simulink model "fan_Ex5"  (R2023b)
settings: Solver=FixedStepAuto  StartTime=0.0  StopTime=10.0  RelTol=1e-3
settings Model: Creator=Fartash  LastModifiedBy=Fartash
settings OptimizationCC: DefaultParameterBehavior=Inlined  EnhancedBackFolding=on  PassReuseOutputArgsAs=Individual arguments  InitFltsAndDblsToZero=on  OptimizeBlockOrder=speed  DifferentSizesBufferReuse=on  OptimizationCustomize=off  EfficientTunableParamExpr=on
settings DebuggingCC: ParameterTunabilityLossMsg=error
settings HardwareCC: ProdLongLongMode=on  TargetLongLongMode=on
settings SFSimCC: MATLABDynamicMemAlloc=off  SimTargetLang=C++
settings RTWCC: Description=Embedded Coder  SystemTargetFile=ert.tlc  GenCodeOnly=on  TemplateMakefile=ert_default_tmf  Toolchain=MinGW64 | CMake/Ninja (64-bit Windows)  BuildConfiguration=Release  TargetLang=C++  GenerateGPUCode=CUDA
settings CodeAppCC: ForceParamTrailComments=on  IgnoreCustomStorageClasses=off  OperatorAnnotations=on  SimulinkDataObjDesc=on  SFDataObjDesc=on  InsertBlockDesc=on
settings ERTTargetCC: TargetLangStandard=C++11 (ISO)  GenerateSampleERTMain=on  CodeInterfacePackaging=Reusable function  InlinedParameterPlacement=NonHierarchical  RootIOFormat=Structure reference  ERTCustomFileTemplate=example_file_process.tlc

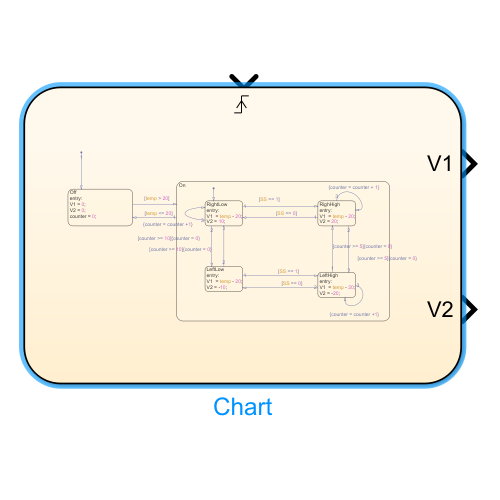
[thumbnail: Simulink's stored preview of the top-level diagram]
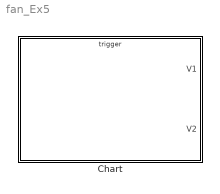
== system fan_Ex5 ==
  Chart : Stateflow chart  TreatAsAtomicUnit=on

== stateflow chart fan_Ex5/Chart ==
  state On
    state RightLow
      entry:
      V1  = temp - 20;
      V2 = 10;
    state RighHigh
      entry:
      V1  = temp - 20;
      V2 = 20;
    state LeftLow
      entry:
      V1  = temp - 20;
      V2 = -10;
    state LeftHigh
      entry:
      V1  = temp - 20;
      V2 = -20;
    (default) -> RightLow
    RighHigh -> RighHigh [order 3] : {counter = counter + 1}
    RightLow -> RighHigh [order 1] : [SS == 1]
    RightLow -> RightLow [order 3] : {counter = counter +1}
    RighHigh -> RightLow [order 1] : [SS == 0]
    RightLow -> LeftLow [order 2] : [counter >= 10]{counter = 0}
    LeftLow -> RightLow [order 2] : [counter >= 10]{counter = 0}
    LeftHigh -> RighHigh [order 1] : [counter >= 5]{counter = 0}
    RighHigh -> LeftHigh [order 2] : [counter >= 5]{counter = 0}
    LeftLow -> LeftHigh [order 1] : [SS == 1]
    LeftHigh -> LeftHigh [order 3] : {counter = counter +1}
    LeftHigh -> LeftLow [order 2] : [SS == 0]
  state Off
    entry:
    V1 = 0;
    V2 = 0;
    counter = 0;
  (default) -> Off
  Off -> On : [temp > 20]
  On -> Off : [temp <= 20]
  data: counter local; V1 output; V2 output
  events: temp input RISING_EDGE_EVENT; SS input RISING_EDGE_EVENT
